simulink model "SmartGrid1"  (R2023a)
settings: Solver=FixedStepDiscrete  StartTime=0.0  StopTime=5  FixedStep=1e-6  RelTol=1e-3
undefined symbols (not defined in the file or in its folder): Ion, Lithium
libraries: spsSeriesRLCBranchLib x6, spsCurrentMeasurementLib x3, spsMosfetLib x2, slpidlib x2, spsVoltageMeasurementLib x2, simulink x1, spsBatteryLib x1, spsPVArrayLib x1, spsDiodeLib x1, spsIGBTDiodeLib x1, spsPWMGeneratorDCDCLib x1, sps_lib x1
settings Model: Creator=Dishan Dey  LastModifiedBy=Dishan Dey

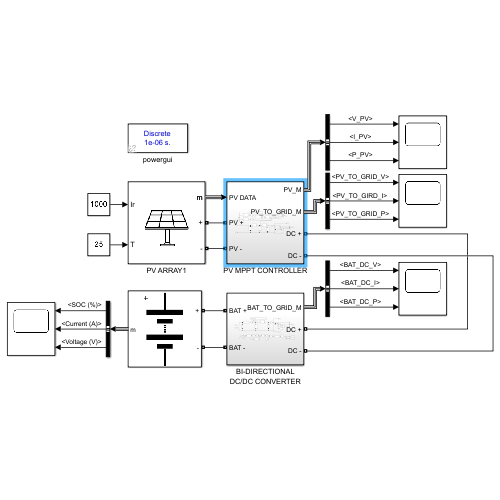
[thumbnail: Simulink's stored preview of the top-level diagram]
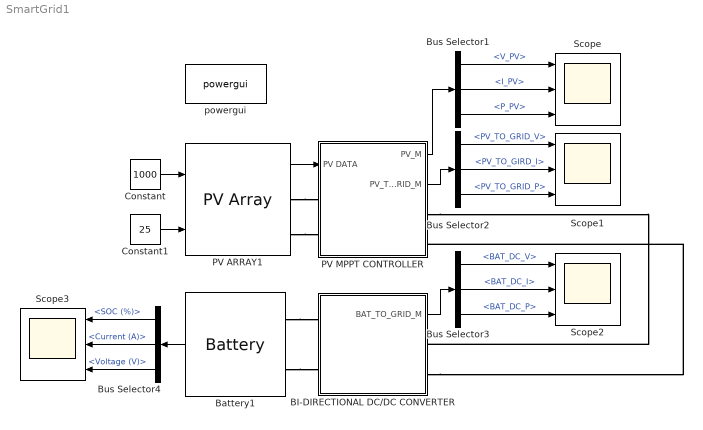
== system SmartGrid1 ==
  BI-DIRECTIONAL DC/DC CONVERTER : Subsystem
  Battery1 : spsBatteryLib/Battery  BatType=Lithium-Ion  ShowTempParam=off  ThermalPreset=no  ShowAgeParam=off  NomV=420  NomQ=600  SOC=80  Batt_Tr=30  PresetModel=on  MaxQ=600  MinV=315  FullV=488.8746  Dis_rate=260.8696  R=0.007  Normal_OP=542.6087  expZone="[453.7621      29.47826]"  current=[6.5 13 32.5]  Units=Time  Tci=20  NomT=20  T2=-30  MaxQ2=4.8  FullV2=7.1  Normal_OP2=5.655  expZone2="[6.58           1]"  Rca=0.6  ti=2000  Dp=0  Neq0=0  Tsim=1e6  Ta1=25  Qeol=5.4*0.9  Reol=0.013333*1.2  Char_age=[2.3478, 3]  Dis_age=[2.3478, 10]  N1=1500  N2=10500  N3=1000  N4=1400  Ta2=45  N5=950
  Bus Selector1 : BusSelector  OutputSignals=V_PV,I_PV,P_PV
  Bus Selector2 : BusSelector  OutputSignals=PV_TO_GRID_V,PV_TO_GIRD_I,PV_TO_GRID_P
  Bus Selector3 : BusSelector  OutputSignals=BAT_DC_V,BAT_DC_I,BAT_DC_P
  Bus Selector4 : BusSelector  OutputSignals=SOC (%),Current (A),Voltage (V)
  Constant : Constant  Value=1000  SampleTime=1e-6
  Constant1 : Constant  Value=25  SampleTime=1e-6
  PV ARRAY1 : spsPVArrayLib/PV Array  Npar=1092  Nser=11  PlotType=array @ 25 deg.C & specified irradiances  S_vec="[ 1000  500  100 ]"  Temp_C_vec="[ 45 25  ]"  ModuleName=Canadian Solar Inc. CS6P-250P  PlotWhenSelected=off  Pm=249.83  Ncell=60  Voc=37.2  Isc=8.87  Vm=30.1  Im=8.3  beta_Voc_pc=-0.301  alpha_Isc_pc=0.038997  beta_Voc=-0.11197  alpha_Isc=0.003459  IL=8.8849  I0=3.0928e-11  nI=0.91537  Rsh=202.8148  Rs=0.34115  RobustModel=off  RobustCellTemperature=313.3991  BAL=on  Tc=1e-6  Tfilter=5e-5
  PV MPPT CONTROLLER : Subsystem
  Scope{,1..3} (4 alike) : Scope  NumInputPorts=3
  powergui : sps_lib/powergui  Priority=1  SimulationMode=Discrete  SampleTime=1e-6  frequency=60  Iterations=50  frequencyindice=0  Pbase=100e6  ErrMax=1e-4  UnitsV=kV  UnitsW=MW  buscounter=0  FunctionMessages=off  echomessages=off  EnableUseOfTLC=off  CurrentSourceSwitches=off  DisableSnubberDevices=off  DisableRonSwitches=off  DisableVfSwitches=off  DisplayEquations=off  AutomaticDiscreteSolvers=off  SolverType=Tustin/Backward Euler (TBE)  Interpol=off  ExternalGateDelay=off  methode=off  Ts=100  x0status=blocks  SPID=on  SwTol=0  HookPort=off  NonlinearTolerance=1e-4  nMaxIteration=100  ContinueOnMaxIteration=off  RestoreLinks=warning  ResistiveCurrentMeasurement=off  Frange=[0:2:500]  Ylog=off  Xlog=on  ShowGrid=off  save=off  variable=ZData  structure=0  ZoomFFT=off  StartTime=0.0  cycles=1  DisplayStyle=1  fundamental=60  FreqAxis=off  MaxFrequency=1000  frequencyindicesteady=1  RmsSteady=1  display=off
  wires:
  PV ARRAY1/1 -> PV MPPT CONTROLLER/1(PV DATA)
  Constant/1 -> PV ARRAY1/1
  Constant1/1 -> PV ARRAY1/2
  PV MPPT CONTROLLER/1(PV_M) -> Bus Selector1/1
  Bus Selector1/1 -> Scope/1  "<V_PV>"
  Bus Selector1/2 -> Scope/2  "<I_PV>"
  Bus Selector1/3 -> Scope/3  "<P_PV>"
  PV MPPT CONTROLLER/2(PV_TO_GRID_M) -> Bus Selector2/1
  Bus Selector2/1 -> Scope1/1  "<PV_TO_GRID_V>"
  Bus Selector2/2 -> Scope1/2  "<PV_TO_GIRD_I>"
  Bus Selector2/3 -> Scope1/3  "<PV_TO_GRID_P>"
  BI-DIRECTIONAL DC/DC CONVERTER/1(BAT_TO_GRID_M) -> Bus Selector3/1
  Bus Selector3/1 -> Scope2/1  "<BAT_DC_V>"
  Bus Selector3/2 -> Scope2/2  "<BAT_DC_I>"
  Bus Selector3/3 -> Scope2/3  "<BAT_DC_P>"
  Battery1/1 -> Bus Selector4/1
  Bus Selector4/1 -> Scope3/1  "<SOC (%)>"
  Bus Selector4/2 -> Scope3/2  "<Current (A)>"
  Bus Selector4/3 -> Scope3/3  "<Voltage (V)>"
  connections:
  Battery1/LConn1 -- BI-DIRECTIONAL DC/DC CONVERTER/LConn1
  Battery1/LConn2 -- BI-DIRECTIONAL DC/DC CONVERTER/LConn2
  PV ARRAY1/RConn1 -- PV MPPT CONTROLLER/LConn1
  PV ARRAY1/RConn2 -- PV MPPT CONTROLLER/LConn2
  PV MPPT CONTROLLER/RConn1 -- BI-DIRECTIONAL DC/DC CONVERTER/RConn1
  BI-DIRECTIONAL DC/DC CONVERTER/RConn2 -- PV MPPT CONTROLLER/RConn2

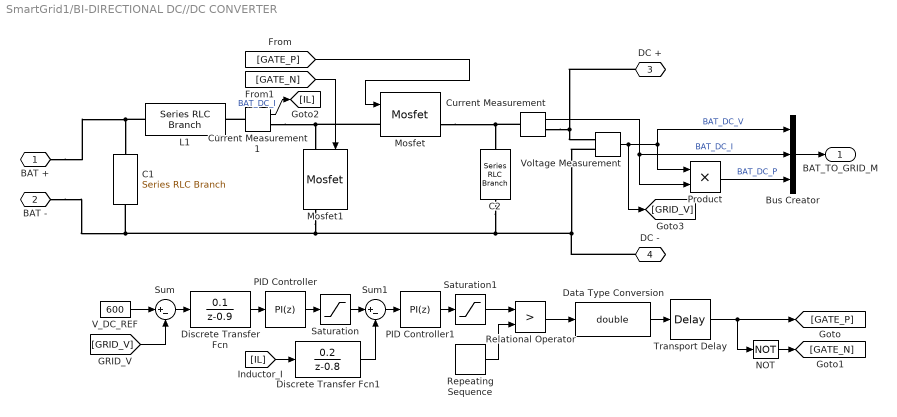
== system SmartGrid1/BI-DIRECTIONAL DC//DC CONVERTER ==
  Bus Creator : BusCreator  Inputs=3
  C1 : spsSeriesRLCBranchLib/Series RLC Branch  LConnTagsString=__new0  RConnTagsString=__new0  BranchType=RC  Resistance=1e-3  Inductance=1e-3  SetiL0=off  InitialCurrent=0  Capacitance=20e-3  Setx0=off  InitialVoltage=0  Measurements=None
  C2 : spsSeriesRLCBranchLib/Series RLC Branch  LConnTagsString=__new0  RConnTagsString=__new0  BranchType=RC  Resistance=0.5e-3  Inductance=1e-3  SetiL0=off  InitialCurrent=0  Capacitance=30e-3  Setx0=off  InitialVoltage=0  Measurements=None
  Current Measurement : spsCurrentMeasurementLib/Current Measurement  PhasorSimulation=off  OutputType=Complex  PSBequivalent=0
  Current Measurement1 : spsCurrentMeasurementLib/Current Measurement  PhasorSimulation=off  OutputType=Complex  PSBequivalent=0
  Data Type Conversion : DataTypeConversion  OutDataTypeStr=double  SaturateOnIntegerOverflow=off  RndMeth=Floor
  Discrete Transfer Fcn : DiscreteTransferFcn  Numerator=[0.1]  Denominator=[1 -0.9]  SampleTime=1e-4
  Discrete Transfer Fcn1 : DiscreteTransferFcn  Numerator=[0.2]  Denominator=[1 -0.8]  SampleTime=1e-4
  L1 : spsSeriesRLCBranchLib/Series RLC Branch  LConnTagsString=__new0  RConnTagsString=__new0  BranchType=RL  Resistance=0.2e-3  Inductance=60e-6  SetiL0=off  InitialCurrent=0  Capacitance=1e-6  Setx0=off  InitialVoltage=0  Measurements=None
  Mosfet : spsMosfetLib/Mosfet  Ron=0.1  Lon=0  Rd=0.01  Vfd=0  IC=0  Rs=1e5  Cs=inf  Measurements=on
  Mosfet1 : spsMosfetLib/Mosfet  Ron=0.1  Lon=0  Rd=0.01  Vfd=0  IC=0  Rs=1e5  Cs=inf  Measurements=on
  NOT : Logic  Operator=NOT  IconShape=distinctive  AllPortsSameDT=off  OutDataTypeStr=boolean
  PID Controller : slpidlib/PID Controller  Controller=PI  Form=Parallel  TimeDomain=Discrete-time  UseExternalTs=off  SampleTime=1e-4  IntegratorMethod=Forward Euler  FilterMethod=Forward Euler  ControllerParametersSource=internal  P=0.002  I=8  UseKiTs=off  D=0  N=100  UseFilter=on  TunerSelectOption=Transfer Function Based (PID Tuner App)  InitialConditionSource=internal  InitialConditionForIntegrator=0  InitialConditionForFilter=0  DifferentiatorICPrevScaledInput=0  ExternalReset=none  TrackingMode=off  Kt=1  LimitOutput=off  SatLimitsSource=internal  UpperSaturationLimit=inf  LowerSaturationLimit=-inf  LinearizeAsGain=on  AntiWindupMode=none  Kb=1  LimitIntegrator=off  UpperIntegratorSaturationLimit=inf  LowerIntegratorSaturationLimit=-inf  POutMin=[]  POutMax=[]  IOutMin=[]  IOutMax=[]  DOutMin=[]  DOutMax=[]  NOutMin=[]  NOutMax=[]  SumOutMin=[]  SumOutMax=[]  SaturationOutMin=[]  SaturationOutMax=[]  PParamMin=[]  PParamMax=[]  IParamMin=[]  IParamMax=[]  DParamMin=[]  DParamMax=[]  NParamMin=[]  NParamMax=[]  KbParamMin=[]  KbParamMax=[]  KtParamMin=[]  KtParamMax=[]  KbOutMin=[]  KbOutMax=[]  KtOutMin=[]  KtOutMax=[]  IntegratorOutMin=[]  IntegratorOutMax=[]  FilterOutMin=[]  FilterOutMax=[]  SumI1OutMin=[]  SumI1OutMax=[]  SumI2OutMin=[]  SumI2OutMax=[]  SumI3OutMin=[]  SumI3OutMax=[]  SumI4OutMin=[]  SumI4OutMax=[]  SumDOutMin=[]  SumDOutMax=[]  DifferentiatorOutMin=[]  DifferentiatorOutMax=[]  FilterDiffOutCoefMin=[]  FilterDiffOutCoefMax=[]  ReciprocalOutMin=[]  ReciprocalOutMax=[]  SumDenOutMin=[]  SumDenOutMax=[]  SumNumOutMin=[]  SumNumOutMax=[]  DivideOutMin=[]  DivideOutMax=[]  UdiffTsProdOutMin=[]  UdiffTsProdOutMax=[]  NTsProdOutMin=[]  NTsProdOutMax=[]  UintegralTsProdOutMin=[]  UintegralTsProdOutMax=[]  UngainTsProdOutMin=[]  UngainTsProdOutMax=[]  ClampingZeroOutDataTypeStr=Inherit: Inherit via back propagation  ClampingZeroOutMin=[]  ClampingZeroOutMax=[]  FilterDenConstantOutDataTypeStr=Inherit: Inherit via back propagation  FilterDenConstantOutMin=[]  FilterDenConstantOutMax=[]  PCopyOutDataTypeStr=Inherit: Inherit via back propagation  PCopyOutMin=[]  PCopyOutMax=[]  NCopyOutDataTypeStr=Inherit: Inherit via back propagation  NCopyOutMin=[]  NCopyOutMax=[]  IntegratorContinuousStateAttributes=''  IntegratorStateMustResolveToSignalObject=off  IntegratorRTWStateStorageClass=Auto  FilterContinuousStateAttributes=''  FilterStateMustResolveToSignalObject=off  FilterRTWStateStorageClass=Auto  ParallelPVariant=InternalParameters  IdealPVariant=Disabled  IVariant=InternalParameters  DVariant=Disabled  IntegratorVariant=Discrete  SatVariant=Disabled  AWVariant=Passthrough  PCopyVariant=Disabled  TRVariant=Disabled  FdbkBlocksVariant=Forward  IdealPFdbkVariant=Disabled  SatFdbkVariant=Disabled  DerivativeFilterVariant=Disabled  NVariant=Disabled  NCopyVariant=Disabled_SignalSpec  FilterICVariant=Disabled  IntegratorICVariant=InternalICs  ExternalResetVariant=Disabled  TRSumVariant=Passthrough  SumFdbkVariant=Disabled  SumVariant=Sum_PI  TsampFilterVariant=InternalTs  TsampNgainVariant=Passthrough  TsampIntegralVariant=Disabled_SignalSpec  ExternalSaturationOutDataTypeStr=Inherit: Same as second input
  PID Controller1 : slpidlib/PID Controller  Controller=PI  Form=Parallel  TimeDomain=Discrete-time  UseExternalTs=off  SampleTime=1e-4  IntegratorMethod=Forward Euler  FilterMethod=Forward Euler  ControllerParametersSource=internal  P=0.01  I=40  UseKiTs=off  D=0  N=100  UseFilter=on  TunerSelectOption=Transfer Function Based (PID Tuner App)  InitialConditionSource=internal  InitialConditionForIntegrator=0  InitialConditionForFilter=0  DifferentiatorICPrevScaledInput=0  ExternalReset=none  TrackingMode=off  Kt=1  LimitOutput=off  SatLimitsSource=internal  UpperSaturationLimit=inf  LowerSaturationLimit=-inf  LinearizeAsGain=on  AntiWindupMode=none  Kb=1  LimitIntegrator=off  UpperIntegratorSaturationLimit=inf  LowerIntegratorSaturationLimit=-inf  POutMin=[]  POutMax=[]  IOutMin=[]  IOutMax=[]  DOutMin=[]  DOutMax=[]  NOutMin=[]  NOutMax=[]  SumOutMin=[]  SumOutMax=[]  SaturationOutMin=[]  SaturationOutMax=[]  PParamMin=[]  PParamMax=[]  IParamMin=[]  IParamMax=[]  DParamMin=[]  DParamMax=[]  NParamMin=[]  NParamMax=[]  KbParamMin=[]  KbParamMax=[]  KtParamMin=[]  KtParamMax=[]  KbOutMin=[]  KbOutMax=[]  KtOutMin=[]  KtOutMax=[]  IntegratorOutMin=[]  IntegratorOutMax=[]  FilterOutMin=[]  FilterOutMax=[]  SumI1OutMin=[]  SumI1OutMax=[]  SumI2OutMin=[]  SumI2OutMax=[]  SumI3OutMin=[]  SumI3OutMax=[]  SumI4OutMin=[]  SumI4OutMax=[]  SumDOutMin=[]  SumDOutMax=[]  DifferentiatorOutMin=[]  DifferentiatorOutMax=[]  FilterDiffOutCoefMin=[]  FilterDiffOutCoefMax=[]  ReciprocalOutMin=[]  ReciprocalOutMax=[]  SumDenOutMin=[]  SumDenOutMax=[]  SumNumOutMin=[]  SumNumOutMax=[]  DivideOutMin=[]  DivideOutMax=[]  UdiffTsProdOutMin=[]  UdiffTsProdOutMax=[]  NTsProdOutMin=[]  NTsProdOutMax=[]  UintegralTsProdOutMin=[]  UintegralTsProdOutMax=[]  UngainTsProdOutMin=[]  UngainTsProdOutMax=[]  ClampingZeroOutDataTypeStr=Inherit: Inherit via back propagation  ClampingZeroOutMin=[]  ClampingZeroOutMax=[]  FilterDenConstantOutDataTypeStr=Inherit: Inherit via back propagation  FilterDenConstantOutMin=[]  FilterDenConstantOutMax=[]  PCopyOutDataTypeStr=Inherit: Inherit via back propagation  PCopyOutMin=[]  PCopyOutMax=[]  NCopyOutDataTypeStr=Inherit: Inherit via back propagation  NCopyOutMin=[]  NCopyOutMax=[]  IntegratorContinuousStateAttributes=''  IntegratorStateMustResolveToSignalObject=off  IntegratorRTWStateStorageClass=Auto  FilterContinuousStateAttributes=''  FilterStateMustResolveToSignalObject=off  FilterRTWStateStorageClass=Auto  ParallelPVariant=InternalParameters  IdealPVariant=Disabled  IVariant=InternalParameters  DVariant=Disabled  IntegratorVariant=Discrete  SatVariant=Disabled  AWVariant=Passthrough  PCopyVariant=Disabled  TRVariant=Disabled  FdbkBlocksVariant=Forward  IdealPFdbkVariant=Disabled  SatFdbkVariant=Disabled  DerivativeFilterVariant=Disabled  NVariant=Disabled  NCopyVariant=Disabled_SignalSpec  FilterICVariant=Disabled  IntegratorICVariant=InternalICs  ExternalResetVariant=Disabled  TRSumVariant=Passthrough  SumFdbkVariant=Disabled  SumVariant=Sum_PI  TsampFilterVariant=InternalTs  TsampNgainVariant=Passthrough  TsampIntegralVariant=Disabled_SignalSpec  ExternalSaturationOutDataTypeStr=Inherit: Same as second input
  Product : Product
  Relational Operator : RelationalOperator  Operator=>  OutDataTypeStr=boolean  RndMeth=Simplest  InputSameDT=off
  Repeating Sequence : simulink/Sources/Repeating Sequence  rep_seq_t=[0 5e-5 1e-4]  rep_seq_y=[0 1 0]
  Saturation : Saturate  UpperLimit=2500  LowerLimit=-2500
  Saturation1 : Saturate  UpperLimit=0.95  LowerLimit=0.05
  Sum : Sum  Inputs=|+-
  Sum1 : Sum  Inputs=|+-
  Transport Delay : TransportDelay  DelayTime=1e-6
  V_DC_REF : Constant  Value=600  SampleTime=1e-6
  Voltage Measurement : spsVoltageMeasurementLib/Voltage Measurement  PhasorSimulation=off  OutputType=Complex  PSBequivalent=0
  BAT + : PMIOPort  Side=Left
  BAT - : PMIOPort  Port=2  Side=Left
  DC + : PMIOPort  Port=3  Side=Right
  DC - : PMIOPort  Port=4  Side=Right
  BAT_TO_GRID_M : Outport
  wires:
  Product/1 -> Bus Creator/3  "BAT_DC_P"
  Bus Creator/1 -> BAT_TO_GRID_M/1
  Voltage Measurement/1 -> [GRID_V], Bus Creator/1, Product/1  "BAT_DC_V"
  Current Measurement/1 -> Product/2, Bus Creator/2  "BAT_DC_I"
  [GATE_P] -> Mosfet/1
  [GATE_N] -> Mosfet1/1
  Current Measurement1/1 -> [IL]  "BAT_DC_I"
  V_DC_REF/1 -> Sum/1
  [GRID_V] -> Sum/2
  Sum/1 -> Discrete Transfer Fcn/1
  Discrete Transfer Fcn/1 -> PID Controller/1
  PID Controller/1 -> Saturation/1
  [IL] -> Discrete Transfer Fcn1/1
  Saturation/1 -> Sum1/1
  Discrete Transfer Fcn1/1 -> Sum1/2
  Sum1/1 -> PID Controller1/1
  PID Controller1/1 -> Saturation1/1
  Saturation1/1 -> Relational Operator/1
  Repeating Sequence/1 -> Relational Operator/2
  NOT/1 -> [GATE_N]
  Relational Operator/1 -> Data Type Conversion/1
  Data Type Conversion/1 -> Transport Delay/1
  Transport Delay/1 -> NOT/1, [GATE_P]
  connections:
  DC -/RConn1 -- Voltage Measurement/LConn2 -- C2/RConn1 -- Mosfet1/RConn1 -- C1/RConn1 -- BAT -/RConn1
  Current Measurement1/RConn1 -- Mosfet/LConn1 -- Mosfet1/LConn1
  L1/RConn1 -- BAT +/RConn1 -- C1/LConn1
  Current Measurement/LConn1 -- Mosfet/RConn1 -- C2/LConn1
  Current Measurement/RConn1 -- DC +/RConn1 -- Voltage Measurement/LConn1
  Current Measurement1/LConn1 -- L1/LConn1

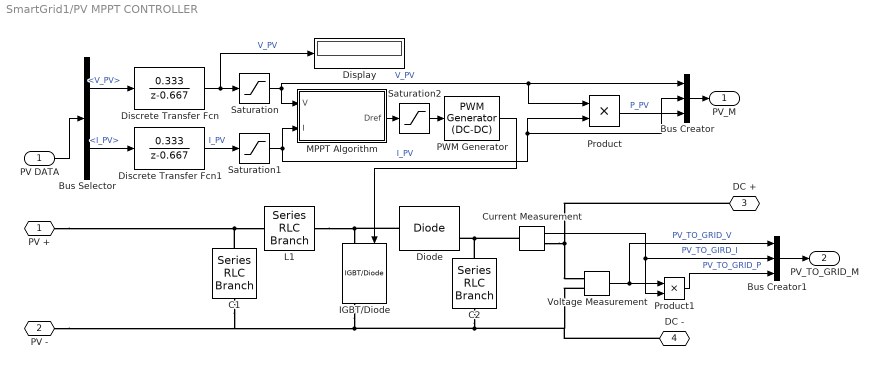
== system SmartGrid1/PV MPPT CONTROLLER ==
  PV DATA : Inport
  Bus Creator : BusCreator  Inputs=3
  Bus Creator1 : BusCreator  Inputs=3
  Bus Selector : BusSelector  OutputSignals=V_PV,I_PV
  C1 : spsSeriesRLCBranchLib/Series RLC Branch  LConnTagsString=__new0  RConnTagsString=__new0  BranchType=RC  Resistance=0.0011  Inductance=1e-3  SetiL0=off  InitialCurrent=0  Capacitance=0.04  Setx0=off  InitialVoltage=0  Measurements=None
  C2 : spsSeriesRLCBranchLib/Series RLC Branch  LConnTagsString=__new0  RConnTagsString=__new0  BranchType=RC  Resistance=0.000004  Inductance=1e-3  SetiL0=off  InitialCurrent=0  Capacitance=0.3  Setx0=off  InitialVoltage=0  Measurements=None
  Current Measurement : spsCurrentMeasurementLib/Current Measurement  PhasorSimulation=off  OutputType=Complex  PSBequivalent=0
  Diode : spsDiodeLib/Diode  Ron=0.001  Lon=0  Vf=0.8  IC=0  UseSnubber=0  Rs=500  Cs=250e-9  Measurements=on
  Discrete Transfer Fcn : DiscreteTransferFcn  Numerator=[0.333]  Denominator=[1 -0.667]  SampleTime=1e-4
  Discrete Transfer Fcn1 : DiscreteTransferFcn  Numerator=[0.333]  Denominator=[1 -0.667]  SampleTime=1e-4
  Display : Display
  IGBT/Diode : spsIGBTDiodeLib/IGBT//Diode  Ron=1e-3  Rs=1e5  Cs=inf  Measurements=on
  L1 : spsSeriesRLCBranchLib/Series RLC Branch  LConnTagsString=__new0  RConnTagsString=__new0  BranchType=L  Resistance=1  Inductance=0.000033  SetiL0=off  InitialCurrent=0  Capacitance=1e-6  Setx0=off  InitialVoltage=0  Measurements=None
  MPPT Algorithm : MATLAB Function  TreatAsAtomicUnit=on
  PWM Generator : spsPWMGeneratorDCDCLib/PWM Generator (DC-DC)  Fsw=10000  Ts=1e-6
  Product : Product
  Product1 : Product
  Saturation : Saturate  UpperLimit=450  LowerLimit=0
  Saturation1 : Saturate  UpperLimit=11000  LowerLimit=0
  Saturation2 : Saturate  UpperLimit=0.44  LowerLimit=0.1
  Voltage Measurement : spsVoltageMeasurementLib/Voltage Measurement  PhasorSimulation=off  OutputType=Complex  PSBequivalent=0
  PV + : PMIOPort  Side=Left
  PV - : PMIOPort  Port=2  Side=Left
  DC + : PMIOPort  Port=3  Side=Right
  DC - : PMIOPort  Port=4  Side=Right
  PV_M : Outport
  PV_TO_GRID_M : Outport  Port=2
  wires:
  PV DATA/1 -> Bus Selector/1
  Product/1 -> Bus Creator/3  "P_PV"
  PWM Generator/1 -> IGBT/Diode/1
  Bus Creator/1 -> PV_M/1
  Bus Creator1/1 -> PV_TO_GRID_M/1
  Voltage Measurement/1 -> Bus Creator1/1, Product1/1  "PV_TO_GRID_V"
  Product1/1 -> Bus Creator1/3  "PV_TO_GRID_P"
  Current Measurement/1 -> Product1/2, Bus Creator1/2  "PV_TO_GIRD_I"
  Bus Selector/1 -> Discrete Transfer Fcn/1  "<V_PV>"
  Discrete Transfer Fcn/1 -> Display/1, Saturation/1  "V_PV"
  Bus Selector/2 -> Discrete Transfer Fcn1/1  "<I_PV>"
  Discrete Transfer Fcn1/1 -> Saturation1/1  "I_PV"
  Saturation/1 -> Product/1, Bus Creator/1, MPPT Algorithm/1(V)  "V_PV"
  Saturation1/1 -> Bus Creator/2, Product/2, MPPT Algorithm/2(I)  "I_PV"
  Saturation2/1 -> PWM Generator/1
  MPPT Algorithm/1(Dref) -> Saturation2/1
  connections:
  PV +/RConn1 -- C1/LConn1 -- L1/RConn1
  L1/LConn1 -- Diode/LConn1 -- IGBT/Diode/LConn1
  IGBT/Diode/RConn1 -- C1/RConn1 -- PV -/RConn1 -- Voltage Measurement/LConn2 -- DC -/RConn1 -- C2/RConn1
  Diode/RConn1 -- Current Measurement/LConn1 -- C2/LConn1
  Current Measurement/RConn1 -- DC +/RConn1 -- Voltage Measurement/LConn1

== matlab function SmartGrid1/PV MPPT CONTROLLER/MPPT Algorithm ==
  settings: updateMethod=DISCRETE
  data: V input; Dref output; I input
function Dref = mppt(V,I)

Dini = 0.45;
Dmax = 0.9;
Dmin = 0.1;
delDref = 0.0005;

persistent Vold Pold Drefold

if isempty(Vold)
    Vold = V;
    Pold = V*I;
    Drefold = Dini;
end

P = V*I;

delV = V - Vold;
delP = P - Pold;

Dref = Drefold;

if delP ~= 0
    if delP > 0
        if delV > 0
            Dref = Drefold - delDref;
        else
            Dref = Drefold + delDref;
        end
    else
        if delV > 0
            Dref = Drefold + delDref;
        else
            Dref = Drefold - delDref;
        end
    end
end

Dref = max(Dmin,min(Dmax,Dref));

Vold = V;
Pold = P;
Drefold = Dref;
